simulink model "quaternionkinematics"  (R2023a)
settings: Solver=VariableStepAuto  StartTime=0.0  StopTime=10.0  RelTol=1e-3
undefined symbols (not defined in the file): pitch, q0, roll, yaw
settings Model: Creator=prafulsigdel  LastModifiedBy=prafulsigdel

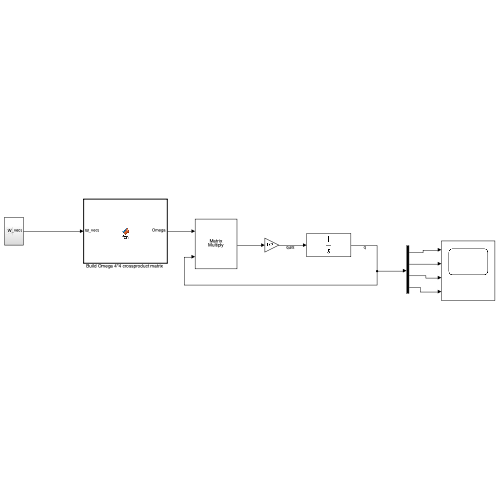
[thumbnail: Simulink's stored preview of the top-level diagram]
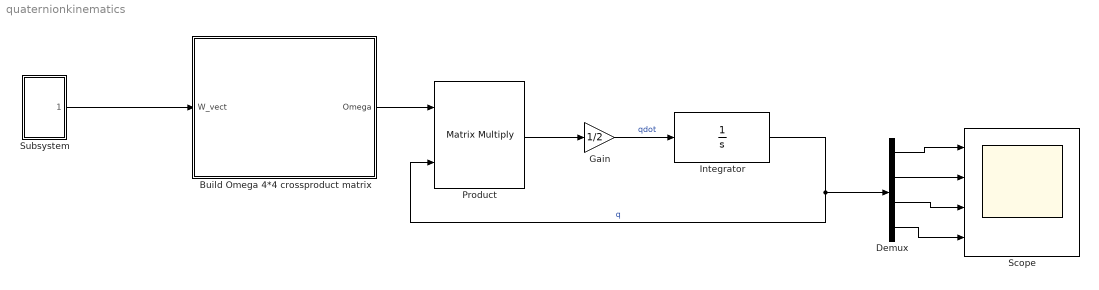
== system quaternionkinematics ==
  "Build Omega 4*4 crossproduct matrix " : MATLAB Function  TreatAsAtomicUnit=on
  Demux : Demux
  Gain : Gain  Gain=1/2
  Integrator : Integrator  InitialCondition=q0
  Product : Product  Multiplication=Matrix(*)
  Scope : Scope  NumInputPorts=4
  Subsystem : Subsystem
  wires:
  Subsystem/1(W_vect) -> "Build Omega 4*4 crossproduct matrix "/1(W_vect)
  "Build Omega 4*4 crossproduct matrix "/1(Omega) -> Product/1
  Integrator/1 -> Product/2, Demux/1  "q"
  Demux/1 -> Scope/1
  Demux/2 -> Scope/2
  Demux/4 -> Scope/4
  Demux/3 -> Scope/3
  Product/1 -> Gain/1
  Gain/1 -> Integrator/1  "qdot"

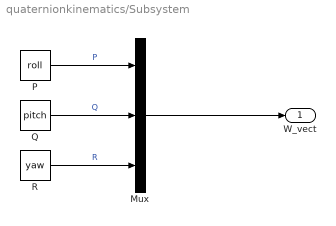
== system quaternionkinematics/Subsystem ==
  Mux : Mux  Inputs=3
  P : Constant  Value=roll
  Q : Constant  Value=pitch
  R : Constant  Value=yaw
  W_vect : Outport
  wires:
  P/1 -> Mux/1  "P"
  R/1 -> Mux/3  "R"
  Q/1 -> Mux/2  "Q"
  Mux/1 -> W_vect/1

== matlab function quaternionkinematics/Build Omega 4*4 crossproduct matrix  ==
  data: W_vect input; Omega output
function Omega = fcn(W_vect)

wx = W_vect(1);
wy = W_vect(2);
wz = W_vect(3);


Omega = [0 -wx -wy -wz;
    wx 0 wz -wy;
    wy -wz 0 wx;
    wz wy -wx 0];
